simulink model "carga_model"  (R2018a)
settings: Solver=FixedStepDiscrete  StartTime=0.0  StopTime=.2  FixedStep=1e-4  MaxStep=1e-5  RelTol=1e-3
InitFcn:
  | Hs = tf([520 0], [1.3801 104 100]);
  | Hz = c2d(Hs, 1e-4, 'impulse');
libraries: simulink_extras x1
settings Model: DataTypeOverride=Off  Creator=erich  LastModifiedBy=erich
settings DataIOCC: SaveOutput=off  SaveTime=off
settings OptimizationCC: BlockReduction=off  ConditionallyExecuteInputs=off  DefaultParameterBehavior=Inlined
settings DebuggingCC: AlgebraicLoopMsg=error  SingleTaskRateTransMsg=error  StrictBusMsg=ErrorOnBusTreatedAsVector
settings HardwareCC: ProdBitPerPointer=32  ProdBitPerSizeT=32  ProdBitPerPtrDiffT=32  ProdLargestAtomicFloat=None  ProdIntDivRoundTo=Undefined  ProdEndianess=Unspecified  ProdWordSize=32  ProdHWDeviceType=ASIC/FPGA->ASIC/FPGA  ProdEqTarget=off
settings CodeAppCC: StateflowObjectComments=on
settings GRTTargetCC: TargetLangStandard=C89/C90 (ANSI)

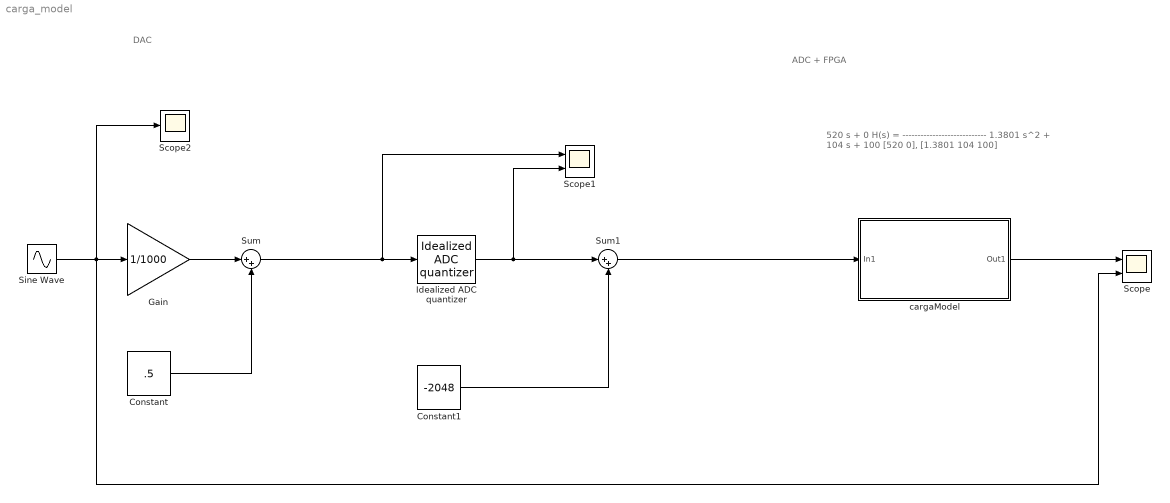
== system carga_model ==
  note: DAC
  note: 520 s  + 0
      | H(s) =    ----------------------------
      | 			1.3801 s^2  +  104 s + 100
      |
      |
      | [520 0], [1.3801 104 100]
  note: ADC + FPGA
  Constant : Constant  Value=.5
  Constant1 : Constant  Value=-2048  OutDataTypeStr=int16
  Gain : Gain  Gain=1/1000
  Idealized ADC quantizer : simulink_extras/Additional Discrete/Idealized ADC quantizer  NumberOfConverterBits=12  Vmin=0  Vmax=1  OutputDataType=int16  OutputNegativeValues=off
      settings: SourceProductName=Simulink
  Scope : Scope  NumInputPorts=2
  Scope1 : Scope  NumInputPorts=2
  Scope2 : Scope
  Sine Wave : Sin  Amplitude=160  Frequency=2*pi*60  SampleTime=1e-4
  Sum : Sum  Inputs=|++
  Sum1 : Sum  Inputs=|++  AccumDataTypeStr=int16  RndMeth=Round
  cargaModel : Subsystem
  wires:
  Sine Wave/1 -> Scope/2, Scope2/1, Gain/1
  Idealized ADC quantizer/1 -> Sum1/1, Scope1/2
  Constant/1 -> Sum/2
  Gain/1 -> Sum/1
  Sum/1 -> Scope1/1, Idealized ADC quantizer/1
  Sum1/1 -> cargaModel/1(In1)
  Constant1/1 -> Sum1/2
  cargaModel/1(Out1) -> Scope/1

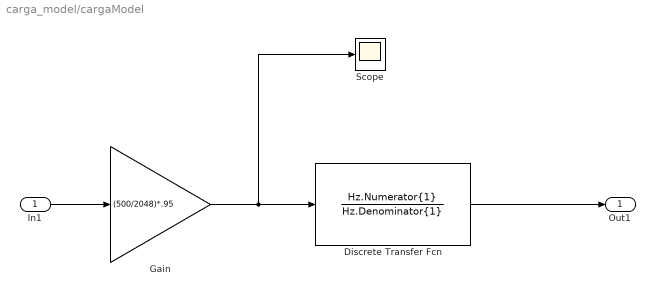
== system carga_model/cargaModel ==
  In1 : Inport
  Discrete Transfer Fcn : DiscreteTransferFcn  Numerator=Hz.Numerator{1}  Denominator=Hz.Denominator{1}  SampleTime=1e-4  StateDataTypeStr=int32  NumCoefDataTypeStr=fixdt(1,32,28)  DenCoefDataTypeStr=fixdt(1,32,28)  NumProductDataTypeStr=fixdt(1,32,10)  DenProductDataTypeStr=fixdt(1,32,10)  NumAccumDataTypeStr=fixdt(1,32,10)  DenAccumDataTypeStr=fixdt(1,32,10)  OutDataTypeStr=int16  RndMeth=Round
  Gain : Gain  Gain=(500/2048)*.95  ParamDataTypeStr=fixdt(1,32,10)
  Scope : Scope
  Out1 : Outport
  wires:
  Discrete Transfer Fcn/1 -> Out1/1
  In1/1 -> Gain/1
  Gain/1 -> Scope/1, Discrete Transfer Fcn/1
